simulink model "model2"  (R2012b)
settings: Solver=ode1  StartTime=0.0  StopTime=inf  FixedStep=0.002  RelTol=1e-3
undefined symbols (not defined in the file or in its folder): HIL
libraries: quarc_library x3
settings Model: SimulationMode=external  ExtModeTrigDuration=500000  Creator=ray.xu  LastModifiedBy=ray.xu
settings SolverCC: PositivePriorityOrder=on
settings RTWCC: SystemTargetFile=quarc_win64.tlc  TemplateMakefile=quarc_default_tmf  Description=QUARC Win64 Target  ProcessScript=quarc_win64_make_rtw_hook
settings STFCustomTargetCC: TargetPreCompLibLocation=C:\PROGRA~3\QUARC\lib\2012b\win64\release  CodeReplacementLibrary=ANSI_C  GeneratePreprocessorConditionals=Disable all  CombineOutputUpdateFcns=on  GRTInterface=off  SystemTargetFile=quarc_win64.tlc
settings GRTTargetCC: TargetPreCompLibLocation=C:\PROGRA~3\QUARC\lib\2012b\win64\release  ParMdlRefBuildCompliant=off  CompOptLevelCompliant=off  ConcurrentExecutionCompliant=off  MatFileLogging=off  ExtMode=on  ExtModeMexFile=quarc_comm
settings ConfigurationSet: Description=SimMechanics 2G

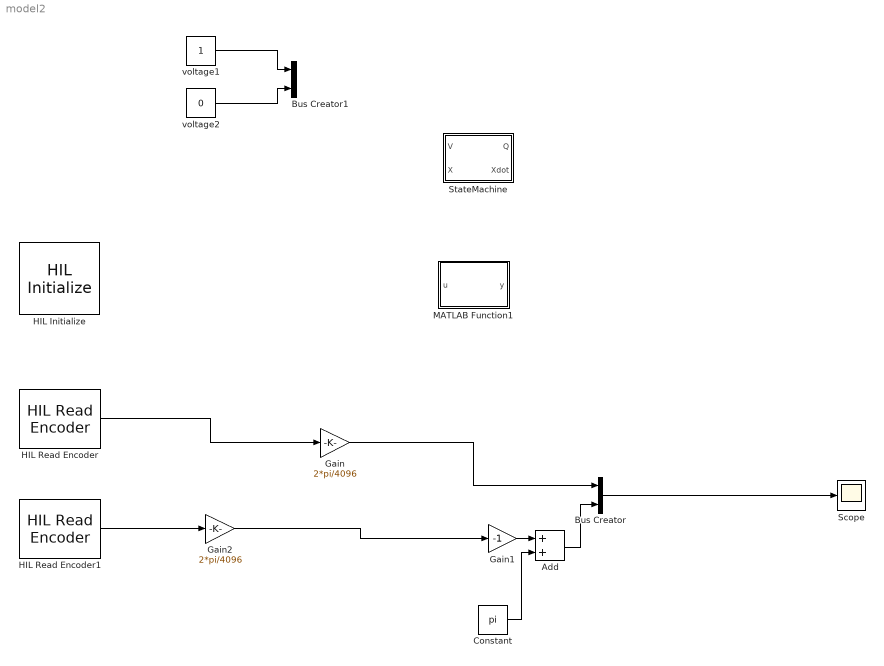
== system model2 ==
  Add : Sum
  Bus Creator : BusCreator  Inputs=2
  Bus Creator1 : BusCreator  Inputs=2
  Constant : Constant  Value=pi
  Gain : Gain  Gain=2*pi/4096
  Gain1 : Gain  Gain=-1
  Gain2 : Gain  Gain=2*pi/4096
  HIL Initialize : quarc_library/Data Acquisition/Generic/Configuration/HIL Initialize  Priority=-99  object_name=HIL-1  board_type=q2_usb  board_number=0  board_options=d0=digital;d1=digital;led=auto;update_rate=normal;decimation=1  exclusive=off  active=off  hardware_clocks=[0]  clock_modes=[]  initial_clock_frequencies=[]  set_clock_params_at_start=off  set_clock_params_at_switch_in=off  set_clock_frequencies_at_start=off  set_clock_frequencies_at_switch_in=off  analog_input_channels=[0:1]  analog_input_maximums=10  analog_input_minimums=-10  set_analog_input_params_at_start=on  set_analog_input_params_at_switch_in=off  analog_output_channels=[0:1]  analog_output_maximums=10  analog_output_minimums=-10  initial_analog_outputs=[0]  final_analog_outputs=[0]  watchdog_analog_outputs=0  set_analog_output_params_at_start=on  set_analog_output_params_at_switch_in=off  set_analog_outputs_at_start=on  set_analog_outputs_at_switch_in=off  set_analog_outputs_at_terminate=on  set_analog_outputs_at_switch_out=off  set_analog_outputs_on_watchdog=off  digital_input_channels=[]  digital_output_channels=[]  digital_output_configuration=[]  initial_digital_outputs=[1]  final_digital_outputs=[1]  watchdog_digital_outputs=[1]  set_digital_output_params_at_start=off  set_digital_output_params_at_switch_in=off  set_digital_outputs_at_start=on  set_digital_outputs_at_switch_in=off  set_digital_outputs_at_terminate=on  set_digital_outputs_at_switch_out=off  set_digital_outputs_on_watchdog=off  encoder_channels=[0:1]  quadrature=[4]  encoder_filter_frequency=[]  initial_encoder_counts=[0]  set_encoder_params_at_start=on  set_encoder_params_at_switch_in=off  set_encoder_counts_at_start=on  set_encoder_counts_at_switch_in=off  pwm_channels=[]  pwm_modes=[0]  pwm_frequency=1/0.020  pwm_configuration=[]  pwm_alignment=[]  pwm_polarity=[]  pwm_leading_deadband=[]  pwm_trailing_deadband=[]  initial_pwm_outputs=[0]  final_pwm_outputs=[0]  watchdog_pwm_outputs=[0]  set_pwm_params_at_start=on  set_pwm_params_at_switch_in=off  set_pwm_outputs_at_start=on  set_pwm_outputs_at_switch_in=off  set_pwm_outputs_at_terminate=on  set_pwm_outputs_at_switch_out=off  set_pwm_outputs_on_watchdog=off  other_output_channels=[]  initial_other_outputs=[]  final_other_outputs=[]  watchdog_other_outputs=[]  set_other_outputs_at_start=off  set_other_outputs_at_switch_in=off  set_other_outputs_at_terminate=off  set_other_outputs_at_switch_out=off  set_other_outputs_on_watchdog=off
  HIL Read Encoder : quarc_library/Data Acquisition/Generic/Immediate I//O/HIL Read Encoder  object_name=HIL-1  channels=0  sample_time=qc_get_step_size  active=on  vector_output=off  data_type_mode=Inherit via back propagation  data_type=double
  HIL Read Encoder1 : quarc_library/Data Acquisition/Generic/Immediate I//O/HIL Read Encoder  object_name=HIL-1  channels=1  sample_time=qc_get_step_size  active=on  vector_output=off  data_type_mode=Inherit via back propagation  data_type=double
  MATLAB Function1 : MATLAB Function  TreatAsAtomicUnit=on
  Scope : Scope
      settings: YMin=-7  YMax=14  SaveName=Theta
  StateMachine : MATLAB Function  TreatAsAtomicUnit=on
  voltage1 : Constant
  voltage2 : Constant  Value=0
  wires:
  Add/1 -> Bus Creator/2
  Gain1/1 -> Add/1
  Constant/1 -> Add/2
  HIL Read Encoder/1 -> Gain/1
  Gain/1 -> Bus Creator/1
  HIL Read Encoder1/1 -> Gain2/1
  Gain2/1 -> Gain1/1
  Bus Creator/1 -> Scope/1
  voltage1/1 -> Bus Creator1/1
  voltage2/1 -> Bus Creator1/2

== matlab function model2/MATLAB Function1 ==
  data: u input; y output
function y = fcn(u)
%#codegen

y = u;

== matlab function model2/StateMachine ==
  data: Q output; V input; Xdot output; X input
function [Q, Xdot] =StateMachine(V, X)

% J1=0.0012;
% m2=0.127;
% l1_l2=0.2;
% l2=0.3;
% lc2=0.15;
% beta1=0.015;
% beta2=0.002;
% Ra=2.6;
% kt=0.00768;
% kv=0.00768;
% kr=70;
% 
% theta1=(J1+m2*l1_l2^2)*Ra/(kr*kt);
% theta2=(m2*l2^2/3)*Ra/(kr*kt);
% theta3=(m2*l1_l2*l2/2)*Ra/(kr*kt);

% theta4=(m2*lc2)*Ra/(kr*kt);
% theta5=beta1*Ra/(kr*kt) + kr*kv;
% theta6=beta2*Ra/(kr*kt);

q1=X(1);
q1dot=X(2);
q2=X(3);
q2dot=X(4);

theta1=0.030372023809524;
theta2=0.018426339285714;
theta3=0.018426339285714;
theta4=0.092131696428571;
theta5=0.610144642857143;
theta6=0.009672619047619;

m11=theta1+theta2*sin(q2)^2;
m12=theta3*cos(q2);
m21=theta3*cos(q2);
m22=theta2;
c11=2*theta2*sin(q2)*cos(q2)+theta5;
c12=-theta3*sin(q2)*q2dot;
c21=-theta2*sin(q2)*cos(q2)*q1dot;
c22=theta6;
f1=0;
f2=0;
g=9.8;
g1=0;
g2=-theta4*g*sin(q2);

M=[m11,m12;m21,m22];
C=[c11,c12;c21,c22];
F=[f1;f2];
G=[g1;g2];
qdot=[q1dot;q2dot];

qdotdot=M\(V-C*qdot-F-G);
Xdot=[q1dot,qdotdot(1),q2dot,qdotdot(2)];
Q=[q1;q2];
end
